simulink model "aMPC_simulink_model"  (R2020b)
settings: Solver=FixedStepAuto  StartTime=0.0  StopTime=sim_time  FixedStep=Ts  RelTol=1e-3
values from neighbouring files (symbols this model uses):
  sim_time = 650    [Model_parameters.m]
  Ts = 0.5    [Model_parameters.m]
libraries: simulink x3
settings Model: Creator=ja  LastModifiedBy=ja

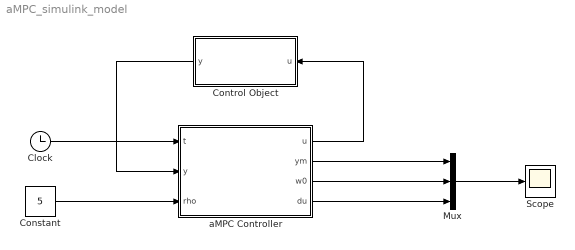
== system aMPC_simulink_model ==
  Clock : Clock
  Constant : Constant  Value=5
  Control Object : Subsystem
  Mux : Mux  Inputs=3
  Scope : Scope
  aMPC Controller : MATLAB Function  TreatAsAtomicUnit=on  SystemSampleTime=Ts
  wires:
  aMPC Controller/1(u) -> Control Object/1(u)
  Control Object/1(y) -> aMPC Controller/2(y)
  Constant/1 -> aMPC Controller/3(rho)
  Clock/1 -> aMPC Controller/1(t)
  aMPC Controller/3(w0) -> Mux/2
  aMPC Controller/2(ym) -> Mux/1
  aMPC Controller/4(du) -> Mux/3
  Mux/1 -> Scope/1

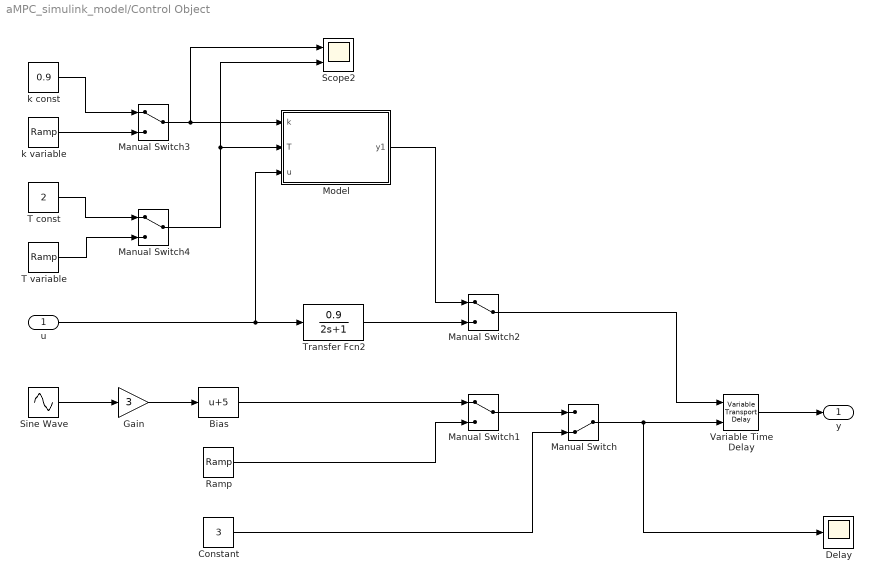
== system aMPC_simulink_model/Control Object ==
  u : Inport
  Bias : Bias  Bias=5
  Constant : Constant  Value=3
  "Delay " : Scope
  Gain : Gain  Gain=3
  Manual Switch : ManualSwitch  CurrentSetting=0
  Manual Switch{1..4} (4 alike) : ManualSwitch
  Model : Subsystem
  Ramp : simulink/Sources/Ramp  slope=6/sim_time  start=0  InitialOutput=2
  Scope2 : Scope  NumInputPorts=2
  Sine Wave : Sin  Frequency=1/100  SampleTime=0
  T const : Constant  Value=2
  T variable : simulink/Sources/Ramp  slope=3/sim_time  start=0  InitialOutput=2
  Transfer Fcn2 : TransferFcn  Numerator=[0.9]  Denominator=[2 1]
  Variable Time Delay : VariableTransportDelay  MaximumDelay=10
  k const : Constant  Value=0.9
  k variable : simulink/Sources/Ramp  slope=4.1/sim_time  start=0  InitialOutput=0.9
  y : Outport
  wires:
  Variable Time Delay/1 -> y/1
  u/1 -> Transfer Fcn2/1, Model/3(u)
  Constant/1 -> Manual Switch/2
  Manual Switch/1 -> "Delay "/1, Variable Time Delay/2
  Manual Switch1/1 -> Manual Switch/1
  Ramp/1 -> Manual Switch1/2
  Sine Wave/1 -> Gain/1
  Gain/1 -> Bias/1
  Bias/1 -> Manual Switch1/1
  Transfer Fcn2/1 -> Manual Switch2/2
  Manual Switch2/1 -> Variable Time Delay/1
  k const/1 -> Manual Switch3/1
  k variable/1 -> Manual Switch3/2
  T const/1 -> Manual Switch4/1
  T variable/1 -> Manual Switch4/2
  Model/1(y1) -> Manual Switch2/1
  Manual Switch3/1 -> Model/1(k), Scope2/1
  Manual Switch4/1 -> Model/2(T), Scope2/2

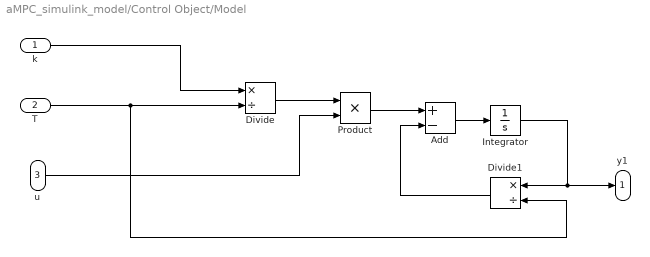
== system aMPC_simulink_model/Control Object/Model ==
  k : Inport
  T : Inport  Port=2
  u : Inport  Port=3
  Add : Sum  Inputs=+-
  Divide : Product  Inputs=*/
  Divide1 : Product  Inputs=*/
  Integrator : Integrator
  Product : Product
  y1 : Outport
  wires:
  Divide1/1 -> Add/2
  Product/1 -> Add/1
  k/1 -> Divide/1
  T/1 -> Divide/2, Divide1/2
  Integrator/1 -> Divide1/1, y1/1
  Add/1 -> Integrator/1
  Divide/1 -> Product/1
  u/1 -> Product/2

== matlab function aMPC_simulink_model/aMPC Controller ==
  data: t input; u output; y input; ym output; w0 output; du output; rho input
function [u, ym ,w0, du] = aMPC(t, y, rho)

    % Persistent variables:
    persistent theta phi du_vec;

    % Variables needed to simulate the model:
    % Simulation time:
    sim_time = 650;
    % Sample time:
    Ts = 0.5;
    % Number of samples:
    n = 50;
    % Prediction horizon:
    H = 25;
    % Control horizon:
    L = 20;

    % Persistent variables initialization:
    if isempty(phi)
        theta = zeros(n, 1);
        phi = zeros(n, 1);
        du_vec = zeros(n, 1);
    end

    %% Parameters estimation algorithm:
    eps = y - phi.' * theta;

    kappa = 1;
    gamma = 1.5 * eye(size(theta, 1));
    m = sqrt(kappa + phi.' * phi);

    % Wyjście z modelu obiektu:
    theta = theta + (gamma * phi * eps / m^2);
    ym = phi.' * theta;

    %% Creating Q matrix:
    Q = zeros(H, L-1);
    for k=1:1:H
        Q(k,1) = theta(k);
    end

    m = 0;
    for j=2:1:L-1
        for k=2:1:H-m
            Q(k+m,j) = Q(k-1,1);
        end
        m = m + 1;
    end

    % Counting sums hj:
    h = zeros(H,1);
    if L >= 2 && H >= L
        for j=1:1:H-L+1
            h(L+j-1) = sum(theta(1:j));
        end
    else
        h = [];
    end
    
    % Matrix Q:
    Q = [Q h];

    %% Reference trajectory:
    traj = [1.0*ones(1,100), 1.5*ones(1,100) 2.0*ones(1,150) 1.0*ones(1,150) 1.5*ones(1,150), 2.0*ones(1,150)];
    w0_d = zeros(H, 1);
    
    for i=1:1:H
        w0_d(i) = traj(floor(t+i*Ts+1));
    end

    %% Incremental predictor:
    y0_d = zeros(H, 1);
    y0_d(1) = y;
    
    for j=2:1:H
        y0_d(j) = y0_d(j-1) + theta(j+1:n)' * du_vec(1:n-j);
    end

    %% Counting vector q:
    T_1 = zeros(L,1); 
    T_1(1) = 1;
    q = (T_1' * (inv(Q' * Q + rho * eye(L))) * Q')';

    %% Counting control signal:
    u = phi(1) + q' * (w0_d - y0_d);

    % Stimulation of the controlled object to start operation aMPC controller:
    if t*1/Ts < 10 
        u=1; 
    end

    % Current control signal increment:
    du = u - phi(1);

    % Updating control signal increments vector:
    du_vec = circshift(du_vec, 1);
    du_vec(1) = du;

    % Update regressor vector:
    phi = circshift(phi, 1);
    phi(1) = u;

    % Current reference trajectory:
    w0 = w0_d(1);

end
